simulink model "PHIL_Load"  (R2016a)
settings: Solver=FixedStepDiscrete  StartTime=0.0  StopTime=15  FixedStep=1e-2  RelTol=1e-3
settings Model: Creator=CoSES_HPC2  LastModifiedBy=CoSES_HPC2
settings DebuggingCC: RootOutportRequireBusObject=error  StrictBusMsg=ErrorOnBusTreatedAsVector
settings HardwareCC: ProdBitPerPointer=32  ProdLargestAtomicFloat=None  ProdWordSize=32  ProdHWDeviceType=Intel->x86/Pentium
settings RTWCC: SystemTargetFile=NIVeriStand.tlc  TemplateMakefile=NIVeriStand_vc.tmf  Description=NI Phar Lap Real-Time & Windows Targets
settings STFCustomTargetCC: MatFileLogging=on  SystemTargetFile=NIVeriStand.tlc
settings GRTTargetCC: ParMdlRefBuildCompliant=off  CompOptLevelCompliant=off  ConcurrentExecutionCompliant=off  GeneratePreprocessorConditionals=Use local settings  CombineOutputUpdateFcns=off  CPPClassGenCompliant=off  GRTInterface=on  UseToolchainInfoCompliant=off

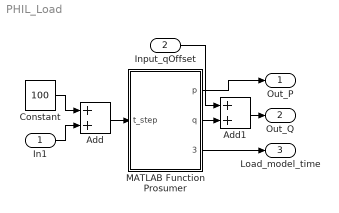
== system PHIL_Load ==
  In1 : Inport
  Input_qOffset : Inport  Port=2
  Add : Sum
  Add1 : Sum
  Constant : Constant  Value=100
  MATLAB Function Prosumer : MATLAB Function  TreatAsAtomicUnit=on
  Out_P : Outport
  Out_Q : Outport  Port=2
  Load_model_time : Outport  Port=3
  wires:
  In1/1 -> Add/2
  MATLAB Function Prosumer/2(q) -> Add1/2
  MATLAB Function Prosumer/1(p) -> Out_P/1
  Add/1 -> MATLAB Function Prosumer/1(t_step)
  Constant/1 -> Add/1
  MATLAB Function Prosumer/3(model_time) -> Load_model_time/1
  Input_qOffset/1 -> Add1/1
  Add1/1 -> Out_Q/1

== matlab function PHIL_Load/MATLAB Function Prosumer ==
  data: p output; q output; t_step input; model_time output
function [p, q, model_time] = fcn(t_step)
persistent counter;

if isempty(counter)
    counter = 0;
end

counter = counter + 1e-2; % in seconds

model_time = counter;
if counter < t_step
    p = 0;
    q = -1400;   % Enable for DVS Scenario
elseif counter < t_step+200
%    p = 5e3;     % Enable for FFR Scenario
    p = -10e3;   % Enable for DVS Scenario
    q = -6.24e3; % Enable for DVS Scenario
else
    p = 0;
    q = -1400;   % Enable for DVS Scenario
end
%q = 0;           % Enable for FFR Scenario
end
